simulink model "zad3_schema22a"  (R2022a)
settings: Solver=FixedStepAuto  StartTime=0.0  StopTime=1400  FixedStep=1  RelTol=1e-3
values from neighbouring files (symbols this model uses):
  Ag = 0.95    [param1.m]
  Gb = 153    [param1.m]
  Ib = 6.5    [param1.m]
  p2 = best_ch(1,end)    [param1.m]
  Sg = Pop(i,2)    [fitness_last.m]    (also in param1.m = 0.03376)
  Si = best_ch(2,end)    [param1.m]
  Td = Pop(i,1)    [fitness_last.m]    (also in param1.m = 39)
  Ti = 45.383    [param1.m]
  Vg = 1.467    [param1.m]
  Vi = 139.094    [param1.m]
undefined symbols (not defined in the file or in its folder): G0, Ki, s1b
settings Model: Creator=johnypi  LastModifiedBy=DFUNDO
settings ModelReferenceCC: EnableRefExpFcnMdlSchedulingChecks=off
settings RTWCC: Description=Generic Real-Time Target

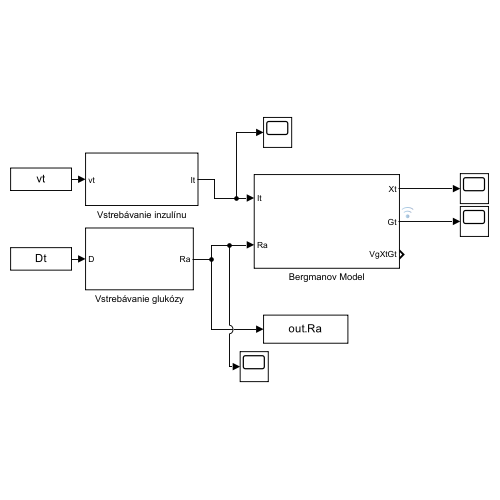
[thumbnail: Simulink's stored preview of the top-level diagram]
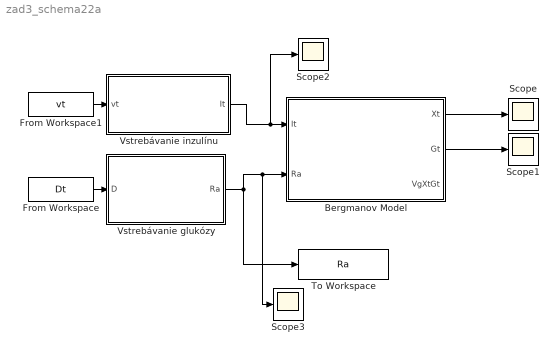
== system zad3_schema22a ==
  Bergmanov Model : Subsystem
  From Workspace : FromWorkspace  VariableName=Dt
  From Workspace1 : FromWorkspace  VariableName=vt
  Scope{,1..3} (4 alike) : Scope
  To Workspace : ToWorkspace  VariableName=Ra  SaveFormat=Timeseries  SampleTime=-1
  Vstrebávanie glukózy : Subsystem
  Vstrebávanie inzulínu : Subsystem
  wires:
  Vstrebávanie inzulínu/1(It) -> Scope2/1, Bergmanov Model/1(It)
  Bergmanov Model/1(Xt) -> Scope/1
  Bergmanov Model/2(Gt) -> Scope1/1
  Vstrebávanie glukózy/1(Ra) -> To Workspace/1, Scope3/1, Bergmanov Model/2(Ra)
  From Workspace/1 -> Vstrebávanie glukózy/1(D)
  From Workspace1/1 -> Vstrebávanie inzulínu/1(vt)

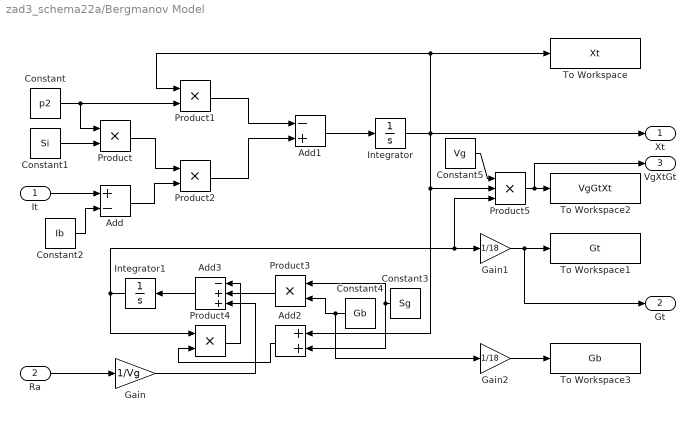
== system zad3_schema22a/Bergmanov Model ==
  It : Inport
  Ra : Inport  Port=2
  Add : Sum  Inputs=+-
  Add1 : Sum  Inputs=-+
  Add2 : Sum
  Add3 : Sum  Inputs=-++
  Constant : Constant  Value=p2
  Constant1 : Constant  Value=Si
  Constant2 : Constant  Value=Ib
  Constant3 : Constant  Value=Sg
  Constant4 : Constant  Value=Gb
  Constant5 : Constant  Value=Vg
  Gain : Gain  Gain=1/Vg
  Gain1 : Gain  Gain=1/18
  Gain2 : Gain  Gain=1/18
  Integrator : Integrator
  Integrator1 : Integrator  InitialCondition=G0
  Product{,1..4} (5 alike) : Product
  Product5 : Product  Inputs=3
  To Workspace : ToWorkspace  VariableName=Xt  SaveFormat=Timeseries  SampleTime=-1
  To Workspace1 : ToWorkspace  VariableName=Gt  SaveFormat=Timeseries  SampleTime=-1
  To Workspace2 : ToWorkspace  VariableName=VgGtXt  SaveFormat=Timeseries  SampleTime=-1
  To Workspace3 : ToWorkspace  VariableName=Gb  SaveFormat=Timeseries  SampleTime=-1
  Xt : Outport
  Gt : Outport  Port=2
  VgXtGt : Outport  Port=3
  wires:
  It/1 -> Add/1
  Add2/1 -> Product4/2
  Constant1/1 -> Product/2
  Product2/1 -> Add1/2
  Ra/1 -> Gain/1
  Add1/1 -> Integrator/1
  Constant4/1 -> Gain2/1, Product3/2
  Product/1 -> Product2/1
  Add/1 -> Product2/2
  Constant2/1 -> Add/2
  Integrator/1 -> Xt/1, Product1/1, To Workspace/1, Product5/2, Add2/1
  Constant3/1 -> Product3/1, Add2/2
  Product1/1 -> Add1/1
  Constant/1 -> Product1/2, Product/1
  Product3/1 -> Add3/2
  Add3/1 -> Integrator1/1
  Product4/1 -> Add3/1
  Gain/1 -> Add3/3
  Integrator1/1 -> Gain1/1, Product5/3, Product4/1
  Constant5/1 -> Product5/1
  Product5/1 -> VgXtGt/1, To Workspace2/1
  Gain1/1 -> Gt/1, To Workspace1/1
  Gain2/1 -> To Workspace3/1

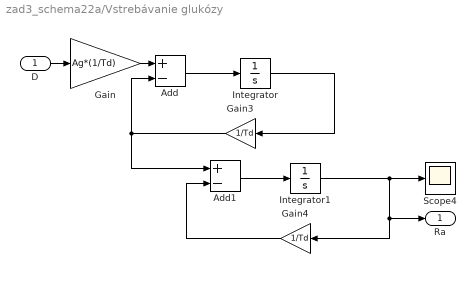
== system zad3_schema22a/Vstrebávanie glukózy ==
  D : Inport
  Add : Sum  Inputs=+-
  Add1 : Sum  Inputs=+-
  Gain : Gain  Gain=Ag*(1/Td)
  Gain3 : Gain  Gain=1/Td
  Gain4 : Gain  Gain=1/Td
  Integrator : Integrator
  Integrator1 : Integrator
  Scope4 : Scope
  Ra : Outport
  wires:
  D/1 -> Gain/1
  Gain4/1 -> Add1/2
  Integrator/1 -> Gain3/1
  Add1/1 -> Integrator1/1
  Gain/1 -> Add/1
  Gain3/1 -> Add1/1, Add/2
  Add/1 -> Integrator/1
  Integrator1/1 -> Scope4/1, Ra/1, Gain4/1

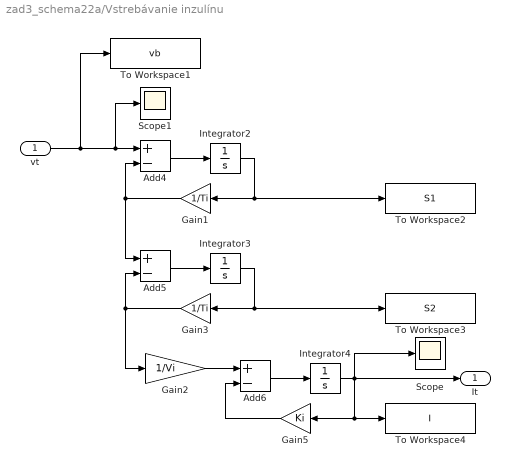
== system zad3_schema22a/Vstrebávanie inzulínu ==
  vt : Inport
  Add4 : Sum  Inputs=+-
  Add5 : Sum  Inputs=+-
  Add6 : Sum  Inputs=+-
  Gain1 : Gain  Gain=1/Ti
  Gain2 : Gain  Gain=1/Vi
  Gain3 : Gain  Gain=1/Ti
  Gain5 : Gain  Gain=Ki
  Integrator2 : Integrator  InitialCondition=s1b
  Integrator3 : Integrator  InitialCondition=s1b
  Integrator4 : Integrator  InitialCondition=Ib
  Scope : Scope
  Scope1 : Scope
  To Workspace1 : ToWorkspace  VariableName=vb  SaveFormat=Timeseries  SampleTime=-1
  To Workspace2 : ToWorkspace  VariableName=S1  SaveFormat=Timeseries  SampleTime=-1
  To Workspace3 : ToWorkspace  VariableName=S2  SaveFormat=Timeseries  SampleTime=-1
  To Workspace4 : ToWorkspace  VariableName=I  SaveFormat=Timeseries  SampleTime=-1
  It : Outport
  wires:
  Integrator2/1 -> To Workspace2/1, Gain1/1
  Add4/1 -> Integrator2/1
  Gain2/1 -> Add6/1
  vt/1 -> To Workspace1/1, Scope1/1, Add4/1
  Gain1/1 -> Add5/1, Add4/2
  Integrator4/1 -> Scope/1, It/1, To Workspace4/1, Gain5/1
  Add5/1 -> Integrator3/1
  Add6/1 -> Integrator4/1
  Integrator3/1 -> To Workspace3/1, Gain3/1
  Gain3/1 -> Gain2/1, Add5/2
  Gain5/1 -> Add6/2
